simulink model "blockdiagrams"  (R2022b)
settings: Solver=VariableStepAuto  StartTime=0.0  StopTime=10.0  RelTol=1e-3
settings Model: Creator=tedbrekken  LastModifiedBy=Bosma
settings ModelReferenceCC: EnableRefExpFcnMdlSchedulingChecks=on

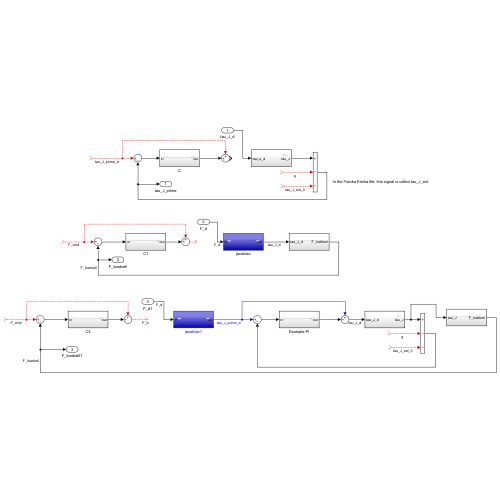
[thumbnail: Simulink's stored preview of the top-level diagram]
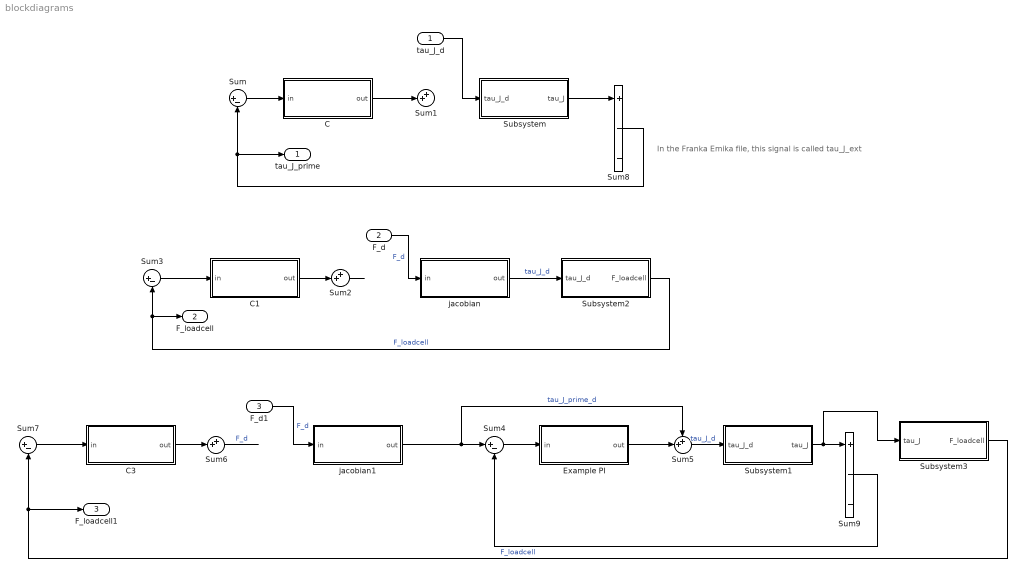
== system blockdiagrams ==
  note: In the Franka Emika file, this signal is called tau_J_ext
  tau_J_d : Inport
  F_d : Inport  Port=2
  F_d1 : Inport  Port=3
  C : Subsystem
  C1 : Subsystem
  C3 : Subsystem
  Example PI : Subsystem
  Subsystem : Subsystem
  Subsystem1 : Subsystem
  Subsystem2 : Subsystem
  Subsystem3 : Subsystem
  Sum{,3..4,7} (4 alike) : Sum  Inputs=|+-
  Sum{1..2,5..6} (4 alike) : Sum  Inputs=++|
  Sum8 : Sum  Inputs=+--
  Sum9 : Sum  Inputs=+--
  jacobian : Subsystem
  jacobian1 : Subsystem
  tau_J_prime : Outport
  F_loadcell : Outport  Port=2
  F_loadcell1 : Outport  Port=3
  wires:
  Sum/1 -> C/1(in)
  C/1(out) -> Sum1/2
  ? -> Sum1/1, Sum/1  "tau_J_prime_d"
  C1/1(out) -> Sum2/2
  jacobian/1(out) -> Subsystem2/1(tau_J_d)  "tau_J_d"
  Sum2/1 -> ?
  Sum3/1 -> C1/1(in)
  ? -> Sum2/1, Sum3/1  "F_cmd"
  Subsystem2/1(F_loadcell) -> F_loadcell/1, Sum3/2  "F_loadcell"
  Sum4/1 -> Example PI/1(in)
  Sum5/1 -> Subsystem1/1(tau_J_d)  "tau_J_d"
  Example PI/1(out) -> Sum5/2
  Sum6/1 -> ?  "F_d"
  jacobian1/1(out) -> Sum5/1, Sum4/1  "tau_J_prime_d"
  Sum9/1 -> Sum4/2
  Sum7/1 -> C3/1(in)
  ? -> Sum6/1, Sum7/1  "F_cmd"
  C3/1(out) -> Sum6/2
  Subsystem3/1(F_loadcell) -> F_loadcell1/1, Sum7/2  "F_loadcell"
  Subsystem/1(tau_J) -> Sum8/1
  ? -> Sum8/2  "g"
  ? -> Sum8/3  "tau_J_ext_0"
  Sum8/1 -> tau_J_prime/1, Sum/2
  tau_J_d/1 -> Subsystem/1(tau_J_d)
  F_d/1 -> jacobian/1(in)  "F_d"
  Subsystem1/1(tau_J) -> Subsystem3/1(tau_J), Sum9/1
  ? -> Sum9/3  "tau_J_ext_0"
  ? -> Sum9/2  "g"
  F_d1/1 -> jacobian1/1(in)  "F_d"

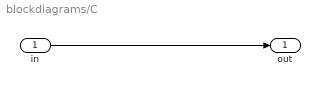
== system blockdiagrams/C ==
  in : Inport
  out : Outport
  wires:
  in/1 -> out/1

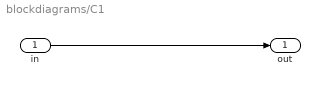
== system blockdiagrams/C1 ==
  in : Inport
  out : Outport
  wires:
  in/1 -> out/1

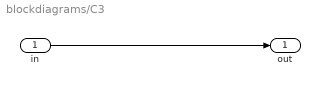
== system blockdiagrams/C3 ==
  in : Inport
  out : Outport
  wires:
  in/1 -> out/1

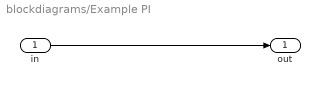
== system blockdiagrams/Example PI ==
  in : Inport
  out : Outport
  wires:
  in/1 -> out/1

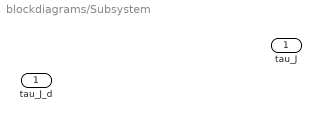
== system blockdiagrams/Subsystem ==
  tau_J_d : Inport
  tau_J : Outport

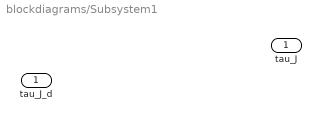
== system blockdiagrams/Subsystem1 ==
  tau_J_d : Inport
  tau_J : Outport

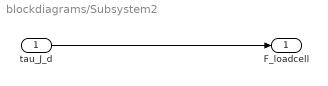
== system blockdiagrams/Subsystem2 ==
  tau_J_d : Inport
  F_loadcell : Outport
  wires:
  tau_J_d/1 -> F_loadcell/1

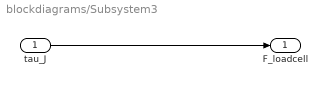
== system blockdiagrams/Subsystem3 ==
  tau_J : Inport
  F_loadcell : Outport
  wires:
  tau_J/1 -> F_loadcell/1

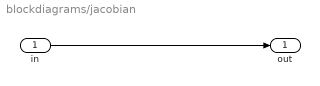
== system blockdiagrams/jacobian ==
  in : Inport
  out : Outport
  wires:
  in/1 -> out/1

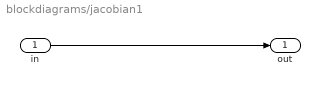
== system blockdiagrams/jacobian1 ==
  in : Inport
  out : Outport
  wires:
  in/1 -> out/1
